simulink model "DRV_Unit"  (R2020b)
settings: configuration reference "unit_config" (kept outside this file)
libraries: simulink_extras x1
settings Model: DataDictionary=Hybrid_vehicle_update.sldd  SimulationMode=accelerator  Creator=Georg  LastModifiedBy=jy
settings ConfigSetRef: SourceName=unit_config

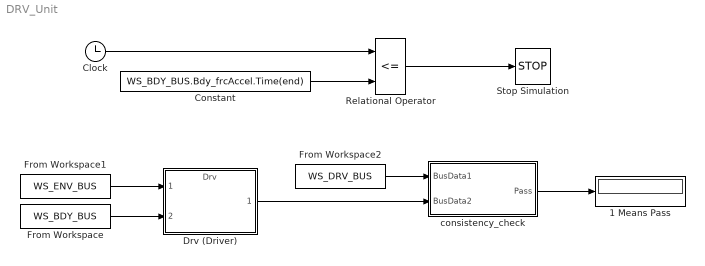
== system DRV_Unit ==
  1 Means Pass : Display
  Clock : Clock
  Constant : Constant  Value=WS_BDY_BUS.Bdy_frcAccel.Time(end)
  Drv (Driver) : ModelReference  ModelNameDialog=Drv  SimulationMode=Normal  ModelReferenceVersion=2.17
      mask Display: image('C:\git\Unit-models-in-Simulink-MIL-tests\updated_structure\img\Driver.jpg'); % Use "Edit Image" on toolstrip to change.
  From Workspace : FromWorkspace  VariableName=WS_BDY_BUS  OutDataTypeStr=Bus: BDY_BUS  SampleTime=0.002  Interpolate=off  OutputAfterFinalValue=Holding final value
  From Workspace1 : FromWorkspace  VariableName=WS_ENV_BUS  OutDataTypeStr=Bus: ENV_BUS  SampleTime=0.002  Interpolate=off  OutputAfterFinalValue=Holding final value
  From Workspace2 : FromWorkspace  VariableName=WS_DRV_BUS  OutDataTypeStr=Bus: DRV_BUS  SampleTime=0.002  Interpolate=off  OutputAfterFinalValue=Holding final value
  Relational Operator : RelationalOperator  Operator=<=  OutDataTypeStr=boolean  RndMeth=Simplest
  Stop Simulation : Stop
  consistency_check : Subsystem
  wires:
  Drv (Driver)/1 -> consistency_check/2(BusData2)
  consistency_check/1(Pass) -> 1 Means Pass/1
  Clock/1 -> Relational Operator/1
  Relational Operator/1 -> Stop Simulation/1
  Constant/1 -> Relational Operator/2
  From Workspace1/1 -> Drv (Driver)/1
  From Workspace/1 -> Drv (Driver)/2
  From Workspace2/1 -> consistency_check/1(BusData1)

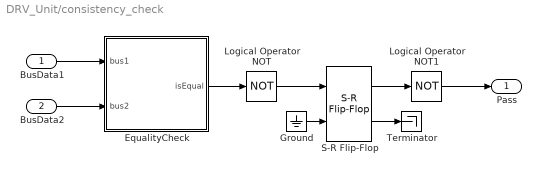
== system DRV_Unit/consistency_check ==
  BusData1 : Inport
  BusData2 : Inport  Port=2
  EqualityCheck : MATLAB Function  TreatAsAtomicUnit=on
  Ground : Ground
  Logical Operator NOT : Logic  Operator=NOT  AllPortsSameDT=off  OutDataTypeStr=boolean
  Logical Operator NOT1 : Logic  Operator=NOT  AllPortsSameDT=off  OutDataTypeStr=boolean
  S-R Flip-Flop : simulink_extras/Flip Flops/S-R Flip-Flop  initial_condition=0
  Terminator : Terminator
  Pass : Outport  VectorParamsAs1DForOutWhenUnconnected=off
  wires:
  BusData1/1 -> EqualityCheck/1(bus1)
  BusData2/1 -> EqualityCheck/2(bus2)
  EqualityCheck/1(isEqual) -> Logical Operator NOT/1
  Logical Operator NOT/1 -> S-R Flip-Flop/1
  Ground/1 -> S-R Flip-Flop/2
  S-R Flip-Flop/2 -> Terminator/1
  S-R Flip-Flop/1 -> Logical Operator NOT1/1
  Logical Operator NOT1/1 -> Pass/1

== matlab function DRV_Unit/consistency_check/EqualityCheck ==
  data: bus1 input; isEqual output; bus2 input
function isEqual = fcn(bus1, bus2)
isEqual = isequal(bus1, bus2);
